simulink model "cruisecontrol"  (R2020b)
settings: Solver=VariableStepAuto  StartTime=0.0  StopTime=120  RelTol=1e-3
values from neighbouring files (symbols this model uses):
  b = 50    [cruisecontrol.mat]
  kd = 1    [cruisecontrol.mat]
  ki = 1    [cruisecontrol.mat]
  Kp = 100    [cruisecontrol.mat]
  m = 1000    [cruisecontrol.mat]
settings Model: Creator=Acer  LastModifiedBy=Acer

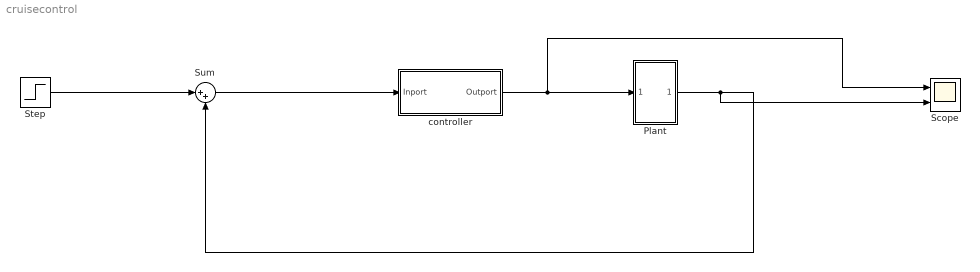
== system cruisecontrol ==
  Plant : Subsystem
  Scope : Scope  NumInputPorts=2
  Step : Step  SampleTime=0
  Sum : Sum  Inputs=|++
  controller : Subsystem
  wires:
  Sum/1 -> controller/1(Inport)
  controller/1(Outport) -> Scope/1, Plant/1(Inport)
  Plant/1(Outport) -> Scope/2, Sum/2
  Step/1 -> Sum/1

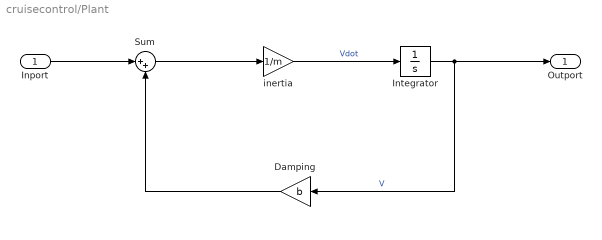
== system cruisecontrol/Plant ==
  Inport : Inport
  Damping : Gain  Gain=b
  Integrator : Integrator
  Sum : Sum  Inputs=|++
  inertia : Gain  Gain=1/m
  Outport : Outport
  wires:
  Sum/1 -> inertia/1
  Integrator/1 -> Outport/1, Damping/1  "V"
  inertia/1 -> Integrator/1  "Vdot"
  Inport/1 -> Sum/1
  Damping/1 -> Sum/2

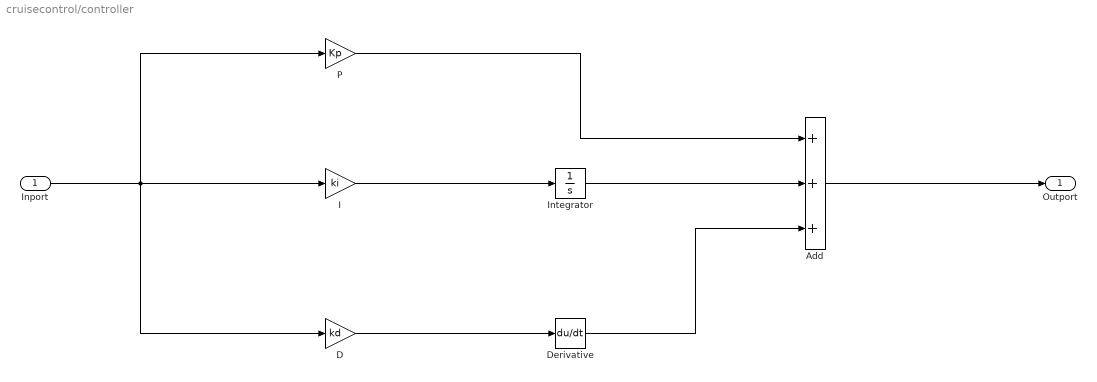
== system cruisecontrol/controller ==
  Inport : Inport
  Add : Sum  Inputs=+++
  D : Gain  Gain=kd
  Derivative : Derivative
  I : Gain  Gain=ki
  Integrator : Integrator
  P : Gain  Gain=Kp
  Outport : Outport
  wires:
  I/1 -> Integrator/1
  D/1 -> Derivative/1
  Integrator/1 -> Add/2
  Derivative/1 -> Add/3
  P/1 -> Add/1
  Inport/1 -> D/1, I/1, P/1
  Add/1 -> Outport/1
